simulink model "AdaptiveHeadlight"  (R2020a)
settings: Solver=VariableStepAuto  StartTime=0.0  StopTime=10.0  RelTol=1e-3
undefined symbols (not defined in the file): sigbuilder_block
libraries: simulink x2, dspsrcs4 x1
settings Model: Creator=Admin  LastModifiedBy=Admin

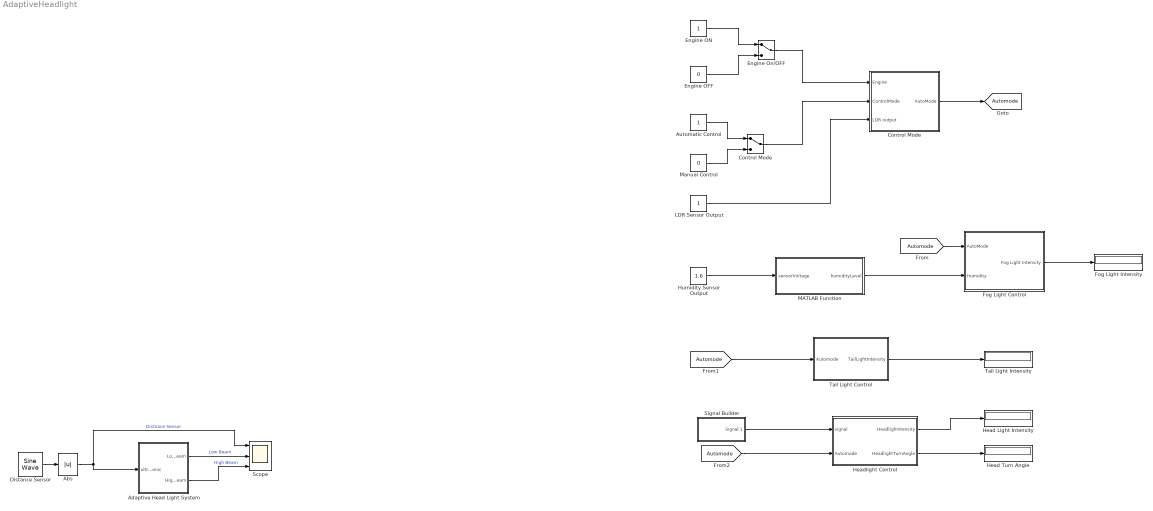
== system AdaptiveHeadlight ==
  " Automatic Control" : Constant
  " Control Mode" : Subsystem
  Abs : Abs
  Adaptive Head Light System : Stateflow chart  TreatAsAtomicUnit=on
  Control Mode : ManualSwitch
  Distance Sensor : dspsrcs4/Sine Wave  Amplitude=7  Frequency=5  Phase=0  SampleMode=Discrete  OutComplex=Real  CompMethod=Trigonometric fcn  TableSize=Speed  SampleTime=1/1000  SamplesPerFrame=1  ResetState=Catch up to simulation time  OutputFrames=off  dataType=double  wordLen=16  udDataType=sfix(16)  fracBitsMode=Best precision  numFracBits=15  OutDataTypeStr=double  LastOutDataTypeStr=double
  Engine OFF : Constant  Value=0
  Engine ON : Constant
  Engine On/OFF : ManualSwitch
  Fog Light Control : Subsystem
  Fog Light Intensity : Display
  Head Light Intensity : Display
  Head Turn Angle : Display
  Headlight Control : Subsystem
  Humidity Sensor Output : Constant  Value=1.6
  LDR Sensor Output : Constant
  MATLAB Function : MATLAB Function  TreatAsAtomicUnit=on
  Manual Control : Constant  Value=0
  Scope : Scope  NumInputPorts=3
  Signal Builder : Subsystem  Tag=STV Subsys  LoadFcn=sigbuilder_block('load');  StartFcn=sigbuilder_block('start');  StopFcn=sigbuilder_block('stop');  ClipboardFcn=sigbuilder_block('clipboard');  mask(Sigbuilder block){tuvar=[0:10]}
      mask help: Simulink:masks:SigbuilderBlock_MD
      mask init:
      | if ~strcmp(get_param(bdroot(gcbh),'SimulationStatus'),'stopped') tuvar = sigbuilder_block('maskInit'); end
      settings: CopyFcn=sigbuilder_block('copy');  DeleteFcn=sigbuilder_block('delete');  ModelCloseFcn=sigbuilder_block('modelClose');  PreSaveFcn=sigbuilder_block('preSave');  PauseFcn=sigbuilder_block('pause');  ContinueFcn=sigbuilder_block('continue');  NameChangeFcn=sigbuilder_block('namechange');  OpenFcn=sigbuilder_block('open',[437.6 199.2 550.4 400 ]);  CloseFcn=sigbuilder_block('close');
      mask Display: plot(0, 0, 100, 100,[2, 2, 32, 32, 2], [68, 8, 8, 68, 68],[32, 2], [38, 38], [32, 19, 2],[53, 60, 44], [32, 17, 17, 2],[16, 16, 31, 31]);txt = getActiveGroup(gcbh);text(2, 100, txt,'verticalAlignment', 'top');
  Tail Light Control : Subsystem
  Tail Light Intensity : Display
  tag scope: Automode=global
  wires:
  Engine ON/1 -> Engine On/OFF/1
  Engine OFF/1 -> Engine On/OFF/2
  Engine On/OFF/1 -> " Control Mode"/1(Engine)
  Control Mode/1 -> " Control Mode"/2(ControlMode)
  Manual Control/1 -> Control Mode/2
  " Automatic Control"/1 -> Control Mode/1
  " Control Mode"/1(AutoMode) -> [Automode]
  Fog Light Control/1(Fog Light Intensity) -> Fog Light Intensity/1
  Humidity Sensor Output/1 -> MATLAB Function/1(sensorVoltage)
  MATLAB Function/1(humidityLevel) -> Fog Light Control/2(Humidity)
  LDR Sensor Output/1 -> " Control Mode"/3(LDR output)
  [Automode] -> Fog Light Control/1(AutoMode)
  [Automode] -> Tail Light Control/1(Automode)
  Tail Light Control/1(TailLightIntensity) -> Tail Light Intensity/1
  [Automode] -> Headlight Control/2(Automode)
  Signal Builder/1(Signal 1) -> Headlight Control/1(signal)
  Headlight Control/1(HeadlighIntensity) -> Head Light Intensity/1
  Headlight Control/2(HeadlightTurnAngle) -> Head Turn Angle/1
  Abs/1 -> Adaptive Head Light System/1(ultrasonic), Scope/1  "Distnace Sensor"
  Distance Sensor/1 -> Abs/1
  Adaptive Head Light System/1(LowBeam) -> Scope/2  "Low Beam"
  Adaptive Head Light System/2(HighBeam) -> Scope/3  "High Beam"

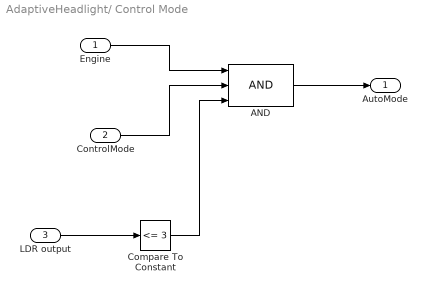
== system AdaptiveHeadlight/ Control Mode ==
  Engine : Inport
  ControlMode : Inport  Port=2
  LDR output : Inport  Port=3
  AND : Logic  Inputs=3  IconShape=distinctive  AllPortsSameDT=off  OutDataTypeStr=boolean
  Compare To Constant : simulink/Logic and Bit Operations/Compare To Constant  relop=<=  const=3  OutDataTypeStr=boolean
  AutoMode : Outport
  wires:
  Engine/1 -> AND/1
  ControlMode/1 -> AND/2
  AND/1 -> AutoMode/1
  LDR output/1 -> Compare To Constant/1
  Compare To Constant/1 -> AND/3

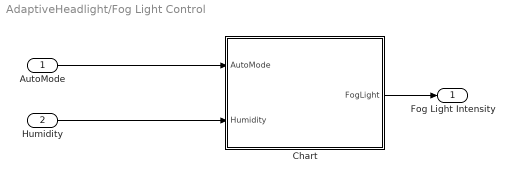
== system AdaptiveHeadlight/Fog Light Control ==
  AutoMode : Inport
  Humidity : Inport  Port=2
  Chart : Stateflow chart  TreatAsAtomicUnit=on
  Fog Light Intensity : Outport
  wires:
  Humidity/1 -> Chart/2(Humidity)
  AutoMode/1 -> Chart/1(AutoMode)
  Chart/1(FogLight) -> Fog Light Intensity/1

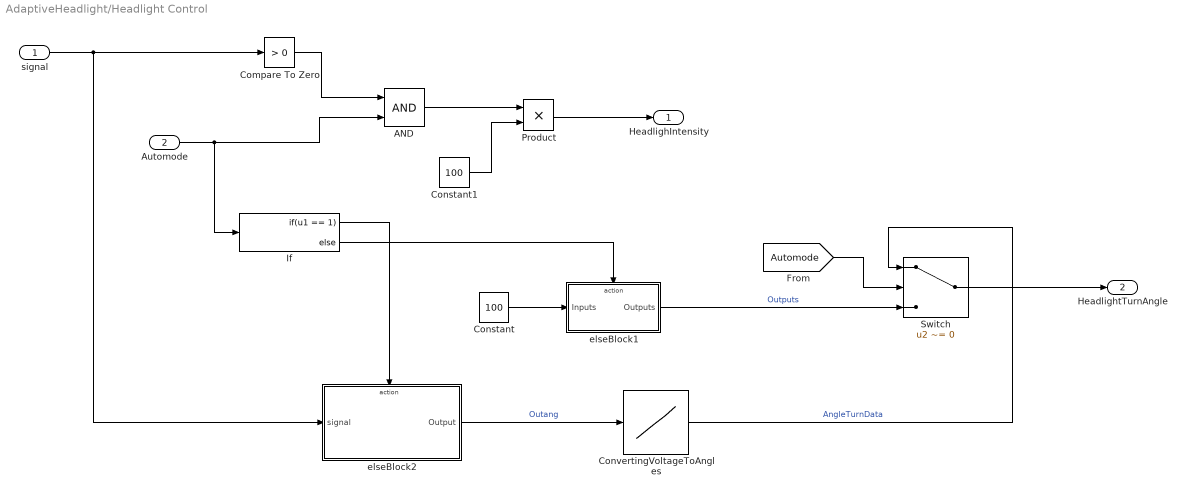
== system AdaptiveHeadlight/Headlight Control ==
  signal : Inport
  Automode : Inport  Port=2
  AND : Logic  IconShape=distinctive  AllPortsSameDT=off  OutDataTypeStr=boolean
  Compare To Zero : simulink/Logic and Bit Operations/Compare To Zero  relop=>  OutDataTypeStr=boolean
  Constant : Constant  Value=100
  Constant1 : Constant  Value=100
  ConvertingVoltageToAngles : Lookup_n-D  NumberOfTableDimensions=1  BreakpointsForDimension1=[0 1 2 3 4 5]  Table=[50 70 90 110 130 150]  ExtrapMethod=Clip  InternalRulePriority=Speed  InputSameDT=on
  If : If  IfExpression=u1 == 1
  Product : Product
  Switch : Switch  Criteria=u2 ~= 0
  elseBlock1 : Subsystem  TreatAsAtomicUnit=on
  elseBlock2 : Subsystem  TreatAsAtomicUnit=on
  HeadlighIntensity : Outport
  HeadlightTurnAngle : Outport  Port=2
  wires:
  signal/1 -> elseBlock2/1(signal), Compare To Zero/1
  AND/1 -> Product/1
  Automode/1 -> If/1, AND/2
  Compare To Zero/1 -> AND/1
  If/1 -> elseBlock2/Action
  If/2 -> elseBlock1/Action
  Constant/1 -> elseBlock1/1(Inputs)
  elseBlock1/1(Outputs) -> Switch/3  "Outputs"
  elseBlock2/1(Output) -> ConvertingVoltageToAngles/1  "Outang"
  ConvertingVoltageToAngles/1 -> Switch/1  "AngleTurnData"
  [Automode] -> Switch/2
  Switch/1 -> HeadlightTurnAngle/1
  Constant1/1 -> Product/2
  Product/1 -> HeadlighIntensity/1

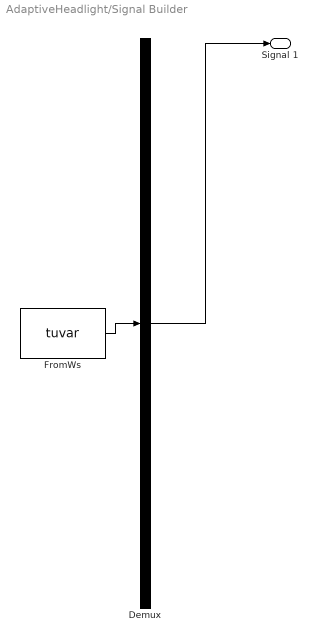
== system AdaptiveHeadlight/Signal Builder ==
  Demux : Demux  Tag=STV Demux  Outputs=1
      settings: DisplayOption=none
  FromWs : FromWorkspace  Tag=STV FromWs  VariableName=tuvar
      SigBuilderData=|
      | common.afterFinalStr = 'Extrapolate'
      | common.sampleTime = 0
      | dataSet.timeRange = [0 10]
      | dataSet.name = 'Group 1'
      | sbobj.Groups.Name = 'Group 1'
      | sbobj.Groups.Signals.Name = 'Signal 1'
      | sbobj.Groups.Signals.XData = [0 4 4 6 6 10]
      | sbobj.Groups.Signals.YData = [0 0 1 1 0 0]
  Signal 1 : Outport  Tag=STV Outport
  wires:
  Demux/1 -> Signal 1/1
  FromWs/1 -> Demux/1

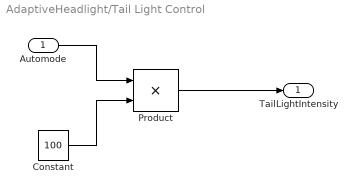
== system AdaptiveHeadlight/Tail Light Control ==
  Automode : Inport
  Constant : Constant  Value=100
  Product : Product
  TailLightIntensity : Outport
  wires:
  Product/1 -> TailLightIntensity/1
  Constant/1 -> Product/2
  Automode/1 -> Product/1

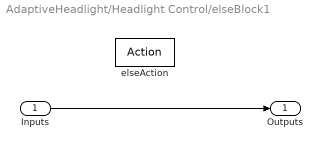
== system AdaptiveHeadlight/Headlight Control/elseBlock1 ==
  Inputs : Inport
  elseAction : ActionPort  ActionPortLabel=else
  Outputs : Outport
  wires:
  Inputs/1 -> Outputs/1

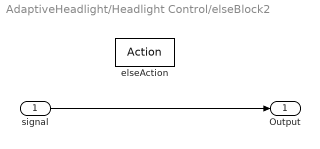
== system AdaptiveHeadlight/Headlight Control/elseBlock2 ==
  signal : Inport
  elseAction : ActionPort  ActionPortLabel=if(u1 == 1)
  Output : Outport
  wires:
  signal/1 -> Output/1

== stateflow chart AdaptiveHeadlight/Adaptive Head Light System ==
  state High_beam
    en: st=1;
    du: HighBeam =1;
    LowBeam =1;
  state Low_decrease
    en: st=2;
    du: HighBeam =0;
    LowBeam =ultrasonic/5;
  state Low_beam
    en: st=3;
    du: HighBeam =0;
    LowBeam =1;
  Low_beam -> High_beam [order 2] : [ultrasonic > 5]
  (default) -> High_beam
  Low_decrease -> High_beam [order 1] : [ultrasonic > 5]
  Low_beam -> Low_decrease [order 1] : [ultrasonic > 0.5 & ultrasonic <=5]
  Low_decrease -> Low_beam [order 2] : [ultrasonic < 0.5]
  High_beam -> Low_decrease [order 1] : [ultrasonic > 0.5 & ultrasonic <=5]
  High_beam -> Low_beam [order 2] : [ultrasonic <= 0.5]
  data: ultrasonic input; LowBeam output; st local; HighBeam output

== matlab function AdaptiveHeadlight/MATLAB Function ==
  data: sensorVoltage input; humidityLevel output
function humidityLevel = fcn(sensorVoltage)

if(sensorVoltage > 0  && sensorVoltage <= 1)
    humidityLevel = 1;                                  %Low humidity, low fog present
elseif(sensorVoltage > 1  && sensorVoltage <= 2)
    humidityLevel = 2;                                  %Medium Humidity, Medium fog present
else
    humidityLevel = 3;                                  %High Humidity, Heavy fog present
end

== stateflow chart AdaptiveHeadlight/Fog Light Control/Chart ==
  (default) -> (junction 25) : % %Fog light intensity control
  (junction 25) -> (junction 26) [order 1] : [AutoMode == 1 && Humidity ==1]
  (junction 25) -> (junction 27) [order 2]
  (junction 26) -> (junction 31) : {FogLight = 30;}
  (junction 27) -> (junction 28) [order 1] : [AutoMode == 1 && Humidity ==2]
  (junction 27) -> (junction 29) [order 2] : {FogLight = 100;}
  (junction 28) -> (junction 30) : {FogLight = 60;}
  (junction 30) -> (junction 29)
  (junction 31) -> (junction 30)
  (junction 29) -> (junction 32)
  data: AutoMode input; Humidity input; FogLight output
